simulink model "UAVFleetNetRead"  (R2013b)
settings: Solver=ode1  StartTime=0.0  StopTime=300  FixedStep=simPars.SampleTime  RelTol=1e-3
libraries: etargetslib x1, instrumentlib x1
settings Model: Creator=Paul Freeman  LastModifiedBy=descobar
settings DataIOCC: LimitDataPoints=off  SignalLoggingSaveFormat=ModelDataLogs  SaveOutput=off  SignalLogging=off
settings OptimizationCC: InlineParams=on  ExpressionDepthLimit=2147483647
settings DebuggingCC: FcnCallInpInsideContextMsg=UseLocalSettings  StateNameClashWarn=warning
settings HardwareCC: ProdLargestAtomicInteger=Long  ProdLargestAtomicFloat=Double  ProdIntDivRoundTo=Zero  ProdEndianess=BigEndian  ProdHWDeviceType=Freescale->32-bit PowerPC
settings SFSimCC: SimParseCustomCode=off
settings GRTTargetCC: CombineOutputUpdateFcns=off  GRTInterface=on

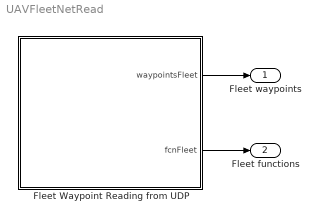
== system UAVFleetNetRead ==
  Fleet Waypoint Reading from UDP : Subsystem
  Fleet waypoints : Outport
  Fleet functions : Outport  Port=2
  wires:
  Fleet Waypoint Reading from UDP/1(waypointsFleet) -> Fleet waypoints/1
  Fleet Waypoint Reading from UDP/2(fcnFleet) -> Fleet functions/1

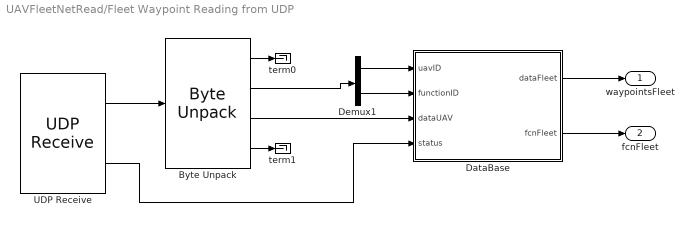
== system UAVFleetNetRead/Fleet Waypoint Reading from UDP ==
  Byte Unpack : etargetslib/Byte Unpack  dimensions={[3],[2],[30], [1]}  datatypes={'uint8', 'uint16', 'double','uint16'}  byteAlign=1
  "DataBase " : MATLAB Function  TreatAsAtomicUnit=on
  Demux1 : Demux  Outputs=2
  UDP Receive : instrumentlib/UDP Receive  Host=localhost  Port=9040  LocalPort=9040  DataSize="[249    1]"  EnableBlockingMode=off  Timeout=10  SampleTime=0.02  DataType=uint8  ByteOrder=BigEndian
  term0 : Terminator
  term1 : Terminator
  waypointsFleet : Outport
  fcnFleet : Outport  Port=2
  wires:
  "DataBase "/1(dataFleet) -> waypointsFleet/1
  Demux1/2 -> "DataBase "/2(functionID)
  UDP Receive/2 -> "DataBase "/4(status)
  Demux1/1 -> "DataBase "/1(uavID)
  Byte Unpack/3 -> "DataBase "/3(dataUAV)
  Byte Unpack/2 -> Demux1/1
  UDP Receive/1 -> Byte Unpack/1
  "DataBase "/2(fcnFleet) -> fcnFleet/1
  Byte Unpack/1 -> term0/1
  Byte Unpack/4 -> term1/1

== matlab function UAVFleetNetRead/Fleet Waypoint Reading from UDP/DataBase  ==
  data: uavID input; functionID input; dataUAV input; dataFleet output; fcnFleet output; status input
function [dataFleet,fcnFleet] = fcn(uavID, functionID , dataUAV, status)
%#codegen
nAC = 2; 
nWPs = 10; % maximum number of waypoints
%argument nAC; 

fcnFleet = zeros(nAC,1) ;

persistent waypointsFleet; 

if isempty(waypointsFleet)
    waypointsFleet = zeros(3,100, nAC);  
end

switch functionID
    case 1 % setting waypoint list of a UAV into database
        if (uavID <= nAC )
            waypointsFleet(:,1:nWPs,uavID) = reshape(dataUAV, 3 ,nWPs  ); 
            if status ==1
                fcnFleet(uavID) =functionID ; % reset
                disp('status = 1') ;
            end
        end
        
        
    otherwise
        
        
    
end


dataFleet = waypointsFleet(1:3,:,:);
